simulink model "sim_three_hop"  (R2020b)
settings: Solver=VariableStepAuto  StartTime=0.0  StopTime=1000  RelTol=1e-3  EnableMultiTasking=on
values from neighbouring files (symbols this model uses):
  sim_vars = [ 1000000, 25                1e-3,                20e3, 5,               20e3, 5,               20e3, 5,               inf, inf, inf                rand(1,1)*100000 ]    [main.m]
undefined symbols (not defined in the file or in its folder): m, n
settings Model: SimulationMode=accelerator  Creator=The MathWorks, Inc.  LastModifiedBy=ssmos
settings DataIOCC: LimitDataPoints=on  SaveOperatingPoint=on  SaveFormat=StructureWithTime
settings OptimizationCC: LifeSpan=inf
settings DebuggingCC: AllowSymbolicDim=off  SFUnexpectedBacktrackingDiag=warning  SFNoUnconditionalDefaultTransitionDiag=warning  SFExecutionAtInitializationDiag=none  ArithmeticOperatorsInVariantConditions=warning
settings ModelReferenceCC: PropagateSignalLabelsOutOfModel=off
settings SFSimCC: SimUseLocalCustomCode=off  CustomCodeUndefinedFunction=UseInterfaceOnly
settings RTWCC: RTWUseLocalCustomCode=off
settings CodeAppCC: StateflowObjectComments=on
settings GRTTargetCC: TargetLangStandard=C89/C90 (ANSI)
settings ConfigComp: CovMetricSettings=dw  CovSaveCumulativeToWorkspaceVar=on  CovSaveSingleToWorkspaceVar=on  CovExternalEMLEnable=off  CovSFcnEnable=off

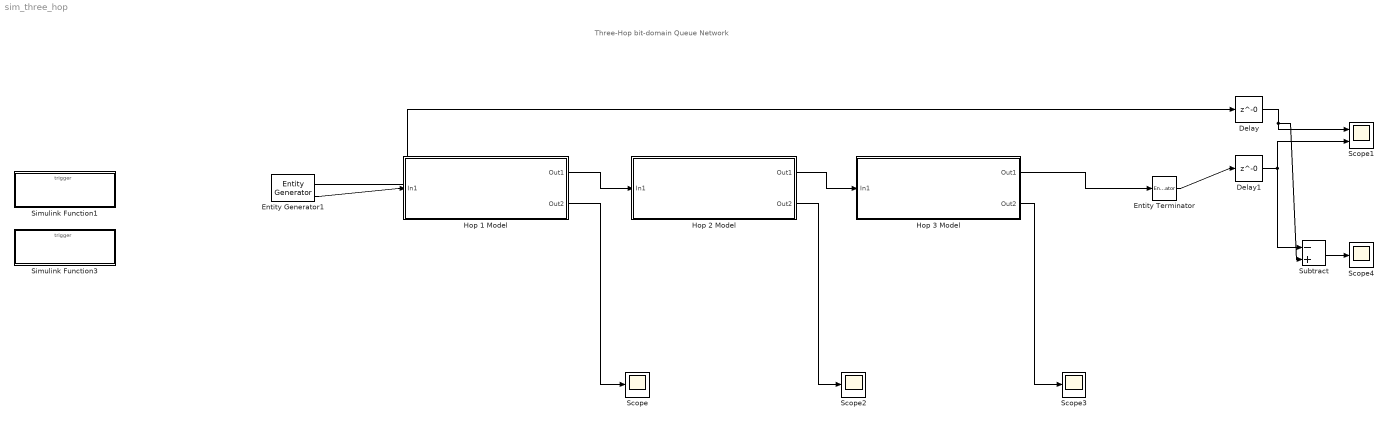
== system sim_three_hop ==
  note: Three-Hop bit-domain Queue Network
  Delay : Delay  DelayLength=0  SampleTime=1
  Delay1 : Delay  DelayLength=0  SampleTime=1
  Entity Generator1 : EntityGenerator  OutputPortMessageModes=n,m  TimeSource=MATLAB action  IntergenerationTimeAction=|  GenerateEntityAtSimulationStart=off  GenerateAction=|  AttributeName=starttime|queuen_uplink_bu|servern_uplink_bu|queuen_compute_bu|servern_compute_bu|queuen_downlink_bu|servern_downlink_bu|queuen_compute_bc|servern_compute_bc|queuen_downlink_bc|servern_downlink_bc|queuen_downlink_bd|servern_downlink_bd|queuetime_uplink|servicetime_uplink|queuetime_compute|servicetime_compute|queuetime_downlink|servicetime_downlink|endtime  AttributeInitialValue=inf|-1|-1|-1|-1|-1|-1|-1|-1|-1|-1|-1|-1|inf|inf|inf|inf|inf|inf|inf  NumberEntitiesDeparted=on  EntityType=Structured  EntityTypeName=Entity
      IntergenerationTimeAction=|
      | T_max = sim_vars(1);
      | rho = sim_vars(2);
      | 
      | persistent T;
      | if isempty(T)
      |     T = 1; 
      | end
      | 
      | persistent next_dt;
      | if isempty(next_dt)
      |     next_dt = 0;
      | end
      | 
      | persistent count igt;
      | if isempty(count)
      |     igt = zeros(1,rho);
      |     igt(end) = 1;
      |     count = 1;
      | end
      | 
      | if T > T_max
      |     dt = inf;
      | else
      |     dt = next_dt;
      |     next_dt = igt(count);
      |     count = count+1;
      |     if (next_dt==1)
      |         count = 1;
      |         T = T + 1;
      |     end
      | end
      GenerateAction=|
      | entity.starttime = getCurrentTime();
      | 
      | entity.queuen_uplink_bu = getQueueNUplink();
      | entity.servern_uplink_bu = getServerNUplink();
      | 
      | entity.queuen_compute_bu = getQueueNCompute();
      | entity.servern_compute_bu = getServerNCompute();
      | 
      | entity.queuen_downlink_bu = getQueueNDownlink();
      | entity.servern_downlink_bu = getServerNDownlink();
      | 
      | %[nd,ne,np] = saveCrossNUplink();
      | %entity.crossn_uplink = nd-ne-np;
      settings: OutputPortMap=o0,o3
  Entity Terminator : EntityTerminator  InputPortMessageModes=m  EntryAction=|  NumberEntitiesArrived=on
      | entity.endtime = getCurrentTime();
      | 
      | saveAttributes([entity.starttime;               ...
      |                 entity.queuen_uplink_bu;        ...
      |                 entity.servern_uplink_bu;       ...
      |                 entity.queuen_compute_bu;       ...
      |                 entity.servern_compute_bu;      ...
      |                 entity.queuen_downlink_bu;      ...
      |                 entity.servern_downlink_bu;     ...
      |                 entity.queuen_compute_bc;       ...
      |                 entity.servern_compute_bc;      ...
      |                 entity.queuen_downlink_bc;      ...
      |                 entity.servern_downlink_bc;     ...
      |                 entity.queuen_downlink_bd;      ...
      |                 entity.servern_downlink_bd;     ...
      |                 entity.queuetime_uplink;        ...
      |                 entity.servicetime_uplink;      ...
      |                 entity.queuetime_compute;       ...
      |                 entity.servicetime_compute;     ...
      |                 entity.queuetime_downlink;      ...
      |                 entity.servicetime_downlink;    ...
      |                 entity.endtime;                 ...
      |                 entitySys.id]);
      settings: OutputPortMap=o0
  Hop 1 Model : Subsystem
  Hop 2 Model : Subsystem
  Hop 3 Model : Subsystem
  Scope{,2..4} (4 alike) : Scope
  Scope1 : Scope  NumInputPorts=2
  Simulink Function1 : Subsystem  TreatAsAtomicUnit=on
  Simulink Function3 : Subsystem  TreatAsAtomicUnit=on
  Subtract : Sum  Inputs=-+
  wires:
  Entity Generator1/2 -> Hop 1 Model/1(In1)
  Hop 2 Model/1(Out1) -> Hop 3 Model/1(In1)
  Entity Generator1/1 -> Delay/1
  Entity Terminator/1 -> Delay1/1
  Delay/1 -> Scope1/1, Subtract/2
  Delay1/1 -> Subtract/1, Scope1/2
  Hop 1 Model/2(Out2) -> Scope/1
  Hop 3 Model/2(Out2) -> Scope3/1
  Hop 2 Model/2(Out2) -> Scope2/1
  Subtract/1 -> Scope4/1
  Hop 3 Model/1(Out1) -> Entity Terminator/1
  Hop 1 Model/1(Out1) -> Hop 2 Model/1(In1)

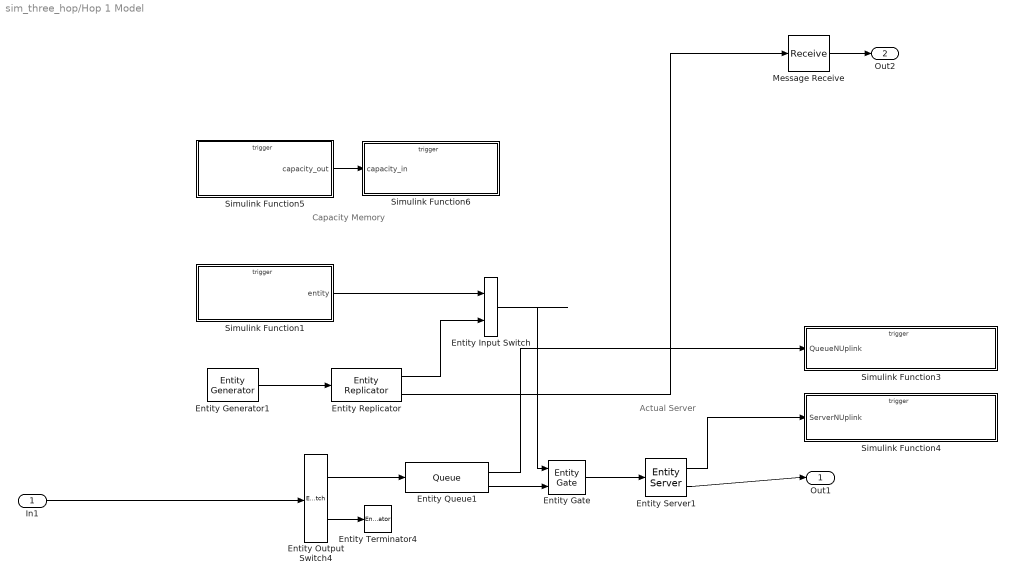
== system sim_three_hop/Hop 1 Model ==
  note: Actual Server
  note: Capacity Memory
  In1 : Inport
  Entity Input Switch : EntityInputSwitch  InputPortMessageModes=m,m  OutputPortMessageModes=m
  Entity Output Switch4 : EntityOutputSwitch  InputPortMessageModes=m  OutputPortMessageModes=m,m  SwitchAttributeName=drop_at_source
  Entity Gate : EntityGate  InputPortMessageModes=m,m  OutputPortMessageModes=m
  Entity Generator1 : EntityGenerator  OutputPortMessageModes=m  TimeSource=MATLAB action  IntergenerationTimeAction=dt = 1;  GenerateAction=|  AttributeName=entity  AttributeInitialValue=0  EntityTypeName=server_capacity_bell
      | time_slot_duration = sim_vars(3);
      | w = sim_vars(4);
      | snr = sim_vars(5);
      | capacity = getServerCapacityHop1(1,time_slot_duration,snr,w,sim_vars(13));
      | capacity_save(capacity);
      | entity = capacity;
  Entity Queue1 : Queue  InputPortMessageModes=m  OutputPortMessageModes=n,m  Capacity=sim_vars(10)  NumberEntitiesInBlock=on
      settings: OutputPortMap=o1,o5
  Entity Replicator : EntityReplicator  InputPortMessageModes=m  OutputPortMessageModes=m,m
  Entity Server1 : EntityServer  InputPortMessageModes=m  OutputPortMessageModes=n,m  Capacity=1  ServiceTimeSource=MATLAB action  ServiceTimeAction=|  EntryAction=|  ServiceCompleteAction=|  NumberEntitiesInBlock=on
      ServiceTimeAction=|
      | capacity = capacity_read();
      | capacity_save(capacity-1);
      | if capacity == 1
      |     close_gate();
      | end
      | dt = 0;
      EntryAction=|
      | % update packet's queue timestamp
      | entity.queuetime_uplink = getCurrentTime();
      ServiceCompleteAction=|
      | % update service time
      | entity.servicetime_uplink = getCurrentTime();
      | 
      | % save network state in front
      | entity.queuen_compute_bc = getQueueNCompute();
      | entity.servern_compute_bc = getServerNCompute();
      | 
      | entity.queuen_downlink_bc = getQueueNDownlink();
      | entity.servern_downlink_bc = getServerNDownlink();
      settings: OutputPortMap=o1,o9
  Entity Terminator4 : EntityTerminator  InputPortMessageModes=m  EntryAction=|
      | saveAttributes([entity.starttime;               ...
      |                 entity.queuen_uplink_bu;        ...
      |                 entity.servern_uplink_bu;       ...
      |                 entity.queuen_compute_bu;       ...
      |                 entity.servern_compute_bu;      ...
      |                 entity.queuen_downlink_bu;      ...
      |                 entity.servern_downlink_bu;     ...
      |                 entity.queuen_compute_bc;       ...
      |                 entity.servern_compute_bc;      ...
      |                 entity.queuen_downlink_bc;      ...
      |                 entity.servern_downlink_bc;     ...
      |                 entity.queuen_downlink_bd;      ...
      |                 entity.servern_downlink_bd;     ...
      |                 entity.queuetime_uplink;        ...
      |                 entity.servicetime_uplink;      ...
      |                 entity.queuetime_compute;       ...
      |                 entity.servicetime_compute;     ...
      |                 entity.queuetime_downlink;      ...
      |                 entity.servicetime_downlink;    ...
      |                 entity.endtime;                 ...
      |                 entitySys.id]);
  Message Receive : Receive  InputPortMessageModes=m  QueueOverwriting=on  QueueLength=1  InitialValue=[0]  SampleTime=1
  Simulink Function1 : Subsystem  TreatAsAtomicUnit=on
  Simulink Function3 : Subsystem  TreatAsAtomicUnit=on
  Simulink Function4 : Subsystem  TreatAsAtomicUnit=on
  Simulink Function5 : Subsystem  TreatAsAtomicUnit=on
  Simulink Function6 : Subsystem  TreatAsAtomicUnit=on
  Out1 : Outport
  Out2 : Outport  Port=2
  wires:
  Entity Queue1/1 -> Simulink Function3/1(QueueNUplink)
  Entity Server1/1 -> Simulink Function4/1(ServerNUplink)
  In1/1 -> Entity Output Switch4/1
  Entity Output Switch4/1 -> Entity Queue1/1
  Entity Output Switch4/2 -> Entity Terminator4/1
  Entity Queue1/2 -> Entity Gate/2
  Entity Gate/1 -> Entity Server1/1
  Simulink Function5/1(capacity_out) -> Simulink Function6/1(capacity_in)
  Entity Server1/2 -> Out1/1
  Simulink Function1/1(entity) -> Entity Input Switch/1
  Entity Input Switch/1 -> Entity Gate/1
  Message Receive/1 -> Out2/1
  Entity Replicator/2 -> Message Receive/1
  Entity Generator1/1 -> Entity Replicator/1
  Entity Replicator/1 -> Entity Input Switch/2

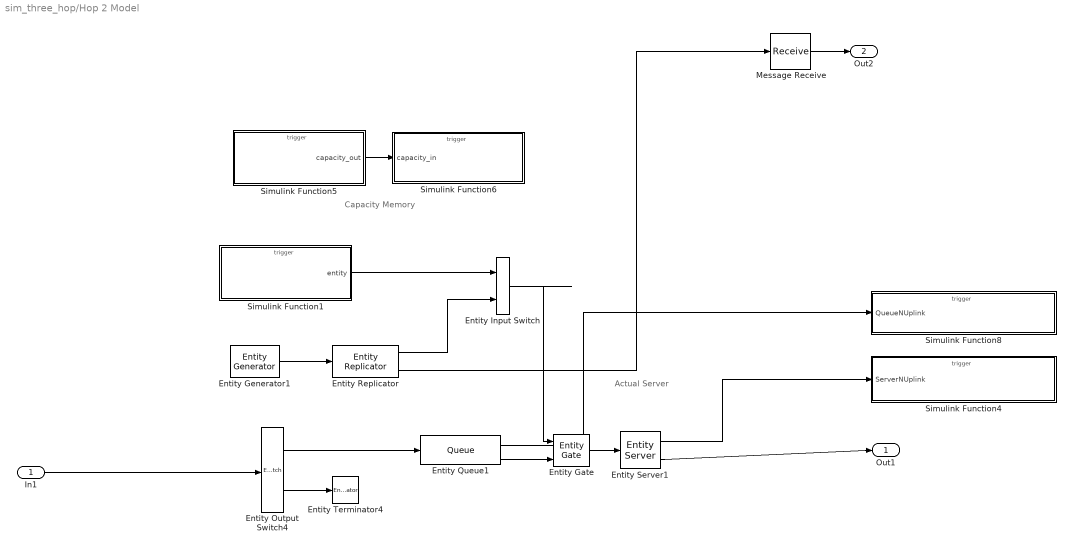
== system sim_three_hop/Hop 2 Model ==
  note: Actual Server
  note: Capacity Memory
  In1 : Inport
  Entity Input Switch : EntityInputSwitch  InputPortMessageModes=m,m  OutputPortMessageModes=m
  Entity Output Switch4 : EntityOutputSwitch  InputPortMessageModes=m  OutputPortMessageModes=m,m  SwitchAttributeName=drop_at_source
  Entity Gate : EntityGate  InputPortMessageModes=m,m  OutputPortMessageModes=m
  Entity Generator1 : EntityGenerator  OutputPortMessageModes=m  TimeSource=MATLAB action  IntergenerationTimeAction=dt = 1;  GenerateAction=|  AttributeName=entity  AttributeInitialValue=0  EntityTypeName=server_capacity_bell
      | time_slot_duration = sim_vars(3);
      | w = sim_vars(6);
      | snr = sim_vars(7);
      | capacity = getServerCapacityHop2(1,time_slot_duration,snr,w,sim_vars(13));
      | capacity_save(capacity);
      | entity = capacity;
  Entity Queue1 : Queue  InputPortMessageModes=m  OutputPortMessageModes=n,m  Capacity=sim_vars(11)  NumberEntitiesInBlock=on
      settings: OutputPortMap=o1,o5
  Entity Replicator : EntityReplicator  InputPortMessageModes=m  OutputPortMessageModes=m,m
  Entity Server1 : EntityServer  InputPortMessageModes=m  OutputPortMessageModes=n,m  Capacity=1  ServiceTimeSource=MATLAB action  ServiceTimeAction=|  EntryAction=|  ServiceCompleteAction=|  NumberEntitiesInBlock=on
      ServiceTimeAction=|
      | capacity = capacity_read();
      | capacity_save(capacity-1);
      | if capacity == 1
      |     close_gate();
      | end
      | dt = 0;
      EntryAction=|
      | % record packet's queue timestamp
      | entity.queuetime_compute = getCurrentTime();
      ServiceCompleteAction=|
      | % record service timestamp
      | entity.servicetime_compute = getCurrentTime();
      | 
      | % record network state in front
      | entity.queuen_downlink_bd = getQueueNDownlink();
      | entity.servern_downlink_bd = getServerNDownlink();
      settings: OutputPortMap=o1,o9
  Entity Terminator4 : EntityTerminator  InputPortMessageModes=m  EntryAction=|
      | saveAttributes([entity.starttime;               ...
      |                 entity.queuen_uplink_bu;        ...
      |                 entity.servern_uplink_bu;       ...
      |                 entity.queuen_compute_bu;       ...
      |                 entity.servern_compute_bu;      ...
      |                 entity.queuen_downlink_bu;      ...
      |                 entity.servern_downlink_bu;     ...
      |                 entity.queuen_compute_bc;       ...
      |                 entity.servern_compute_bc;      ...
      |                 entity.queuen_downlink_bc;      ...
      |                 entity.servern_downlink_bc;     ...
      |                 entity.queuen_downlink_bd;      ...
      |                 entity.servern_downlink_bd;     ...
      |                 entity.queuetime_uplink;        ...
      |                 entity.servicetime_uplink;      ...
      |                 entity.queuetime_compute;       ...
      |                 entity.servicetime_compute;     ...
      |                 entity.queuetime_downlink;      ...
      |                 entity.servicetime_downlink;    ...
      |                 entity.endtime;                 ...
      |                 entitySys.id]);
  Message Receive : Receive  InputPortMessageModes=m  QueueOverwriting=on  QueueLength=1  InitialValue=[0]  SampleTime=1
  Simulink Function1 : Subsystem  TreatAsAtomicUnit=on
  Simulink Function4 : Subsystem  TreatAsAtomicUnit=on
  Simulink Function5 : Subsystem  TreatAsAtomicUnit=on
  Simulink Function6 : Subsystem  TreatAsAtomicUnit=on
  Simulink Function8 : Subsystem  TreatAsAtomicUnit=on
  Out1 : Outport
  Out2 : Outport  Port=2
  wires:
  Entity Queue1/1 -> Simulink Function8/1(QueueNUplink)
  Entity Server1/1 -> Simulink Function4/1(ServerNUplink)
  In1/1 -> Entity Output Switch4/1
  Entity Output Switch4/1 -> Entity Queue1/1
  Entity Server1/2 -> Out1/1
  Entity Output Switch4/2 -> Entity Terminator4/1
  Entity Input Switch/1 -> Entity Gate/1
  Simulink Function1/1(entity) -> Entity Input Switch/1
  Entity Queue1/2 -> Entity Gate/2
  Entity Gate/1 -> Entity Server1/1
  Simulink Function5/1(capacity_out) -> Simulink Function6/1(capacity_in)
  Entity Replicator/2 -> Message Receive/1
  Entity Generator1/1 -> Entity Replicator/1
  Entity Replicator/1 -> Entity Input Switch/2
  Message Receive/1 -> Out2/1

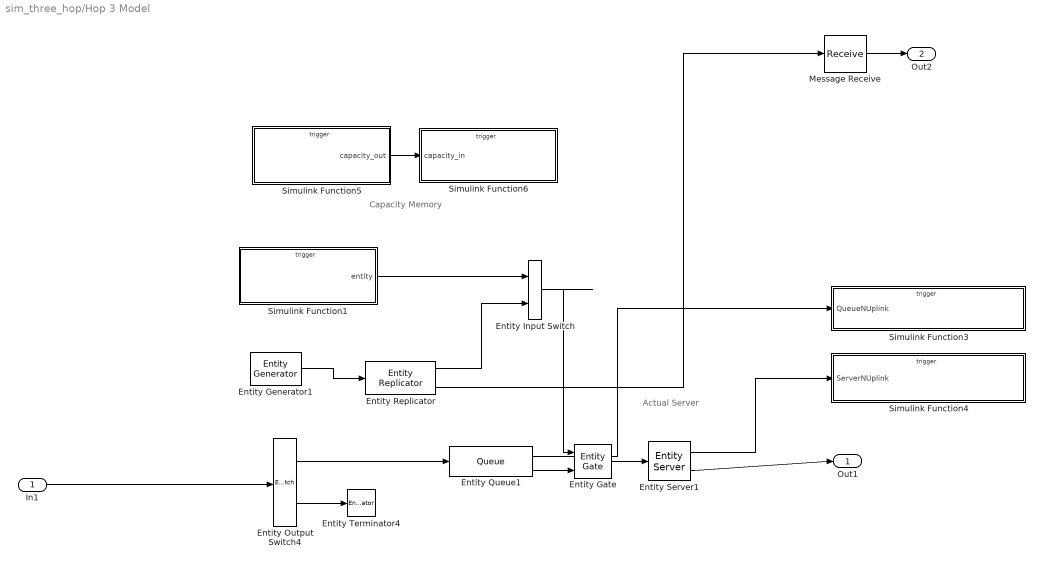
== system sim_three_hop/Hop 3 Model ==
  note: Actual Server
  note: Capacity Memory
  In1 : Inport
  Entity Input Switch : EntityInputSwitch  InputPortMessageModes=m,m  OutputPortMessageModes=m
  Entity Output Switch4 : EntityOutputSwitch  InputPortMessageModes=m  OutputPortMessageModes=m,m  SwitchAttributeName=drop_at_source
  Entity Gate : EntityGate  InputPortMessageModes=m,m  OutputPortMessageModes=m
  Entity Generator1 : EntityGenerator  OutputPortMessageModes=m  TimeSource=MATLAB action  IntergenerationTimeAction=dt = 1;  GenerateAction=|  AttributeName=entity  AttributeInitialValue=0  EntityTypeName=server_capacity_bell
      | time_slot_duration = sim_vars(3);
      | w = sim_vars(8);
      | snr = sim_vars(9);
      | capacity = getServerCapacityHop3(1,time_slot_duration,snr,w,sim_vars(13));
      | capacity_save(capacity);
      | entity = capacity;
  Entity Queue1 : Queue  InputPortMessageModes=m  OutputPortMessageModes=n,m  Capacity=sim_vars(12)  NumberEntitiesInBlock=on
      settings: OutputPortMap=o1,o5
  Entity Replicator : EntityReplicator  InputPortMessageModes=m  OutputPortMessageModes=m,m
  Entity Server1 : EntityServer  InputPortMessageModes=m  OutputPortMessageModes=n,m  Capacity=1  ServiceTimeSource=MATLAB action  ServiceTimeAction=|  EntryAction=|  ServiceCompleteAction=|  NumberEntitiesInBlock=on
      ServiceTimeAction=|
      | capacity = capacity_read();
      | capacity_save(capacity-1);
      | if capacity == 1
      |     close_gate();
      | end
      | dt = 0;
      EntryAction=|
      | % record packet's queue timestamp
      | entity.queuetime_downlink = getCurrentTime();
      ServiceCompleteAction=|
      | % record service timestamp
      | entity.servicetime_downlink = getCurrentTime();
      settings: OutputPortMap=o1,o9
  Entity Terminator4 : EntityTerminator  InputPortMessageModes=m  EntryAction=|
      | saveAttributes([entity.starttime;               ...
      |                 entity.queuen_uplink_bu;        ...
      |                 entity.servern_uplink_bu;       ...
      |                 entity.queuen_compute_bu;       ...
      |                 entity.servern_compute_bu;      ...
      |                 entity.queuen_downlink_bu;      ...
      |                 entity.servern_downlink_bu;     ...
      |                 entity.queuen_compute_bc;       ...
      |                 entity.servern_compute_bc;      ...
      |                 entity.queuen_downlink_bc;      ...
      |                 entity.servern_downlink_bc;     ...
      |                 entity.queuen_downlink_bd;      ...
      |                 entity.servern_downlink_bd;     ...
      |                 entity.queuetime_uplink;        ...
      |                 entity.servicetime_uplink;      ...
      |                 entity.queuetime_compute;       ...
      |                 entity.servicetime_compute;     ...
      |                 entity.queuetime_downlink;      ...
      |                 entity.servicetime_downlink;    ...
      |                 entity.endtime;                 ...
      |                 entitySys.id]);
  Message Receive : Receive  InputPortMessageModes=m  QueueOverwriting=on  QueueLength=1  InitialValue=[0]  SampleTime=1
  Simulink Function1 : Subsystem  TreatAsAtomicUnit=on
  Simulink Function3 : Subsystem  TreatAsAtomicUnit=on
  Simulink Function4 : Subsystem  TreatAsAtomicUnit=on
  Simulink Function5 : Subsystem  TreatAsAtomicUnit=on
  Simulink Function6 : Subsystem  TreatAsAtomicUnit=on
  Out1 : Outport
  Out2 : Outport  Port=2
  wires:
  Entity Queue1/1 -> Simulink Function3/1(QueueNUplink)
  Entity Server1/1 -> Simulink Function4/1(ServerNUplink)
  Entity Output Switch4/1 -> Entity Queue1/1
  Entity Server1/2 -> Out1/1
  Entity Output Switch4/2 -> Entity Terminator4/1
  In1/1 -> Entity Output Switch4/1
  Entity Input Switch/1 -> Entity Gate/1
  Simulink Function5/1(capacity_out) -> Simulink Function6/1(capacity_in)
  Simulink Function1/1(entity) -> Entity Input Switch/1
  Entity Queue1/2 -> Entity Gate/2
  Entity Gate/1 -> Entity Server1/1
  Message Receive/1 -> Out2/1
  Entity Replicator/2 -> Message Receive/1
  Entity Generator1/1 -> Entity Replicator/1
  Entity Replicator/1 -> Entity Input Switch/2

== system sim_three_hop/Simulink Function1 ==
  f : TriggerPort  TriggerType=function-call  IsSimulinkFunction=on  FunctionName=getCurrentTime  VariantControl=(inherit)
  Digital Clock : DigitalClock  SampleTime=-1
  y : ArgOut  DisableCoverage=on  ArgumentName=y
  wires:
  Digital Clock/1 -> y/1

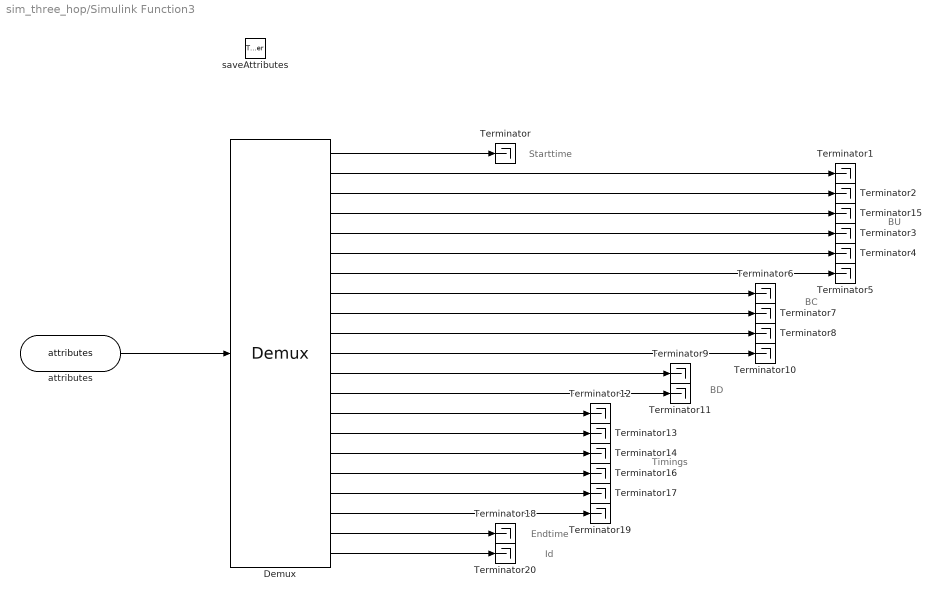
== system sim_three_hop/Simulink Function3 ==
  note: Id
  note: Endtime
  note: Starttime
  note: Timings
  note: BU
  note: BC
  note: BD
  saveAttributes : TriggerPort  TriggerType=function-call  IsSimulinkFunction=on  FunctionName=saveAttributes  VariantControl=(inherit)
  Demux : Demux  Outputs=21
      settings: DisplayOption=none
  Terminator{,1..20} (21 alike) : Terminator
  attributes : ArgIn  DisableCoverage=on  PortDimensions=21  ArgumentName=attributes
  wires:
  attributes/1 -> Demux/1
  Demux/1 -> Terminator/1
  Demux/2 -> Terminator1/1
  Demux/3 -> Terminator2/1
  Demux/7 -> Terminator5/1
  Demux/5 -> Terminator3/1
  Demux/6 -> Terminator4/1
  Demux/8 -> Terminator6/1
  Demux/4 -> Terminator15/1
  Demux/9 -> Terminator7/1
  Demux/10 -> Terminator8/1
  Demux/11 -> Terminator10/1
  Demux/12 -> Terminator9/1
  Demux/13 -> Terminator11/1
  Demux/14 -> Terminator12/1
  Demux/15 -> Terminator13/1
  Demux/16 -> Terminator14/1
  Demux/17 -> Terminator16/1
  Demux/18 -> Terminator17/1
  Demux/19 -> Terminator19/1
  Demux/20 -> Terminator18/1
  Demux/21 -> Terminator20/1

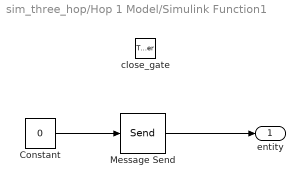
== system sim_three_hop/Hop 1 Model/Simulink Function1 ==
  close_gate : TriggerPort  TriggerType=function-call  IsSimulinkFunction=on  FunctionName=close_gate  FunctionVisibility=scoped  VariantControl=(inherit)
  Constant : Constant  Value=0
  Message Send : Send  OutputPortMessageModes=m
  entity : Outport  InitialOutput=[0]  VectorParamsAs1DForOutWhenUnconnected=off
  wires:
  Message Send/1 -> entity/1
  Constant/1 -> Message Send/1

== system sim_three_hop/Hop 1 Model/Simulink Function3 ==
  QueueNUplink : Inport
  getQueueNUplink : TriggerPort  TriggerType=function-call  IsSimulinkFunction=on  FunctionName=getQueueNUplink  VariantControl=(inherit)
  QueueNCompute : ArgOut  DisableCoverage=on  ArgumentName=QueueNUplink
  wires:
  QueueNUplink/1 -> QueueNCompute/1

== system sim_three_hop/Hop 1 Model/Simulink Function4 ==
  ServerNUplink : Inport
  getServerNUplink : TriggerPort  TriggerType=function-call  IsSimulinkFunction=on  FunctionName=getServerNUplink  VariantControl=(inherit)
  QueueNCompute : ArgOut  DisableCoverage=on  ArgumentName=ServerNUplink
  wires:
  ServerNUplink/1 -> QueueNCompute/1

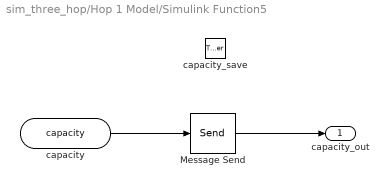
== system sim_three_hop/Hop 1 Model/Simulink Function5 ==
  capacity_save : TriggerPort  TriggerType=function-call  IsSimulinkFunction=on  FunctionName=capacity_save  FunctionVisibility=scoped  VariantControl=(inherit)
  Message Send : Send  OutputPortMessageModes=m
  capacity : ArgIn  DisableCoverage=on  ArgumentName=capacity
  capacity_out : Outport  InitialOutput=[0]  VectorParamsAs1DForOutWhenUnconnected=off
  wires:
  capacity/1 -> Message Send/1
  Message Send/1 -> capacity_out/1

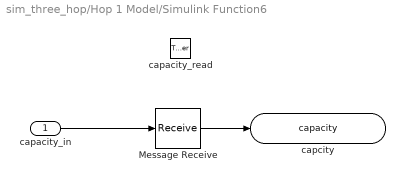
== system sim_three_hop/Hop 1 Model/Simulink Function6 ==
  capacity_in : Inport
  capacity_read : TriggerPort  TriggerType=function-call  IsSimulinkFunction=on  FunctionName=capacity_read  FunctionVisibility=scoped  VariantControl=(inherit)
  Message Receive : Receive  InputPortMessageModes=m  QueueOverwriting=on  QueueLength=1  InitialValue=[0]
  capcity : ArgOut  DisableCoverage=on  ArgumentName=capacity
  wires:
  capacity_in/1 -> Message Receive/1
  Message Receive/1 -> capcity/1

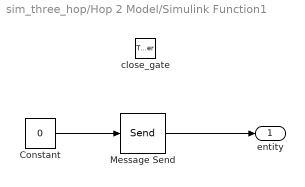
== system sim_three_hop/Hop 2 Model/Simulink Function1 ==
  close_gate : TriggerPort  TriggerType=function-call  IsSimulinkFunction=on  FunctionName=close_gate  FunctionVisibility=scoped  VariantControl=(inherit)
  Constant : Constant  Value=0
  Message Send : Send  OutputPortMessageModes=m
  entity : Outport  InitialOutput=[0]  VectorParamsAs1DForOutWhenUnconnected=off
  wires:
  Message Send/1 -> entity/1
  Constant/1 -> Message Send/1

== system sim_three_hop/Hop 2 Model/Simulink Function4 ==
  ServerNUplink : Inport
  getServerNCompute : TriggerPort  TriggerType=function-call  IsSimulinkFunction=on  FunctionName=getServerNCompute  VariantControl=(inherit)
  ServerNCompute : ArgOut  DisableCoverage=on  ArgumentName=ServerNCompute
  wires:
  ServerNUplink/1 -> ServerNCompute/1

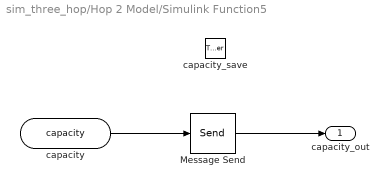
== system sim_three_hop/Hop 2 Model/Simulink Function5 ==
  capacity_save : TriggerPort  TriggerType=function-call  IsSimulinkFunction=on  FunctionName=capacity_save  FunctionVisibility=scoped  VariantControl=(inherit)
  Message Send : Send  OutputPortMessageModes=m
  capacity : ArgIn  DisableCoverage=on  ArgumentName=capacity
  capacity_out : Outport  InitialOutput=[0]  VectorParamsAs1DForOutWhenUnconnected=off
  wires:
  capacity/1 -> Message Send/1
  Message Send/1 -> capacity_out/1

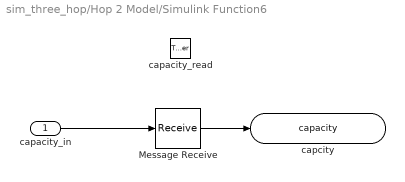
== system sim_three_hop/Hop 2 Model/Simulink Function6 ==
  capacity_in : Inport
  capacity_read : TriggerPort  TriggerType=function-call  IsSimulinkFunction=on  FunctionName=capacity_read  FunctionVisibility=scoped  VariantControl=(inherit)
  Message Receive : Receive  InputPortMessageModes=m  QueueOverwriting=on  QueueLength=1  InitialValue=[0]
  capcity : ArgOut  DisableCoverage=on  ArgumentName=capacity
  wires:
  capacity_in/1 -> Message Receive/1
  Message Receive/1 -> capcity/1

== system sim_three_hop/Hop 2 Model/Simulink Function8 ==
  QueueNUplink : Inport
  getQueueNCompute : TriggerPort  TriggerType=function-call  IsSimulinkFunction=on  FunctionName=getQueueNCompute  VariantControl=(inherit)
  QueueNCompute : ArgOut  DisableCoverage=on  ArgumentName=QueueNCompute
  wires:
  QueueNUplink/1 -> QueueNCompute/1

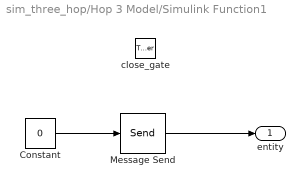
== system sim_three_hop/Hop 3 Model/Simulink Function1 ==
  close_gate : TriggerPort  TriggerType=function-call  IsSimulinkFunction=on  FunctionName=close_gate  FunctionVisibility=scoped  VariantControl=(inherit)
  Constant : Constant  Value=0
  Message Send : Send  OutputPortMessageModes=m
  entity : Outport  InitialOutput=[0]  VectorParamsAs1DForOutWhenUnconnected=off
  wires:
  Message Send/1 -> entity/1
  Constant/1 -> Message Send/1

== system sim_three_hop/Hop 3 Model/Simulink Function3 ==
  QueueNUplink : Inport
  saveQueueNDownlink : TriggerPort  TriggerType=function-call  IsSimulinkFunction=on  FunctionName=getQueueNDownlink  VariantControl=(inherit)
  QueueNDownlink : ArgOut  DisableCoverage=on  ArgumentName=QueueNDownlink
  wires:
  QueueNUplink/1 -> QueueNDownlink/1

== system sim_three_hop/Hop 3 Model/Simulink Function4 ==
  ServerNUplink : Inport
  saveServerNDownlink : TriggerPort  TriggerType=function-call  IsSimulinkFunction=on  FunctionName=getServerNDownlink  VariantControl=(inherit)
  ServerNDownlink : ArgOut  DisableCoverage=on  ArgumentName=ServerNDownlink
  wires:
  ServerNUplink/1 -> ServerNDownlink/1

== system sim_three_hop/Hop 3 Model/Simulink Function5 ==
  capacity_save : TriggerPort  TriggerType=function-call  IsSimulinkFunction=on  FunctionName=capacity_save  FunctionVisibility=scoped  VariantControl=(inherit)
  Message Send : Send  OutputPortMessageModes=m
  capacity : ArgIn  DisableCoverage=on  ArgumentName=capacity
  capacity_out : Outport  InitialOutput=[0]  VectorParamsAs1DForOutWhenUnconnected=off
  wires:
  capacity/1 -> Message Send/1
  Message Send/1 -> capacity_out/1

== system sim_three_hop/Hop 3 Model/Simulink Function6 ==
  capacity_in : Inport
  capacity_read : TriggerPort  TriggerType=function-call  IsSimulinkFunction=on  FunctionName=capacity_read  FunctionVisibility=scoped  VariantControl=(inherit)
  Message Receive : Receive  InputPortMessageModes=m  QueueOverwriting=on  QueueLength=1  InitialValue=[0]
  capcity : ArgOut  DisableCoverage=on  ArgumentName=capacity
  wires:
  capacity_in/1 -> Message Receive/1
  Message Receive/1 -> capcity/1
